simulink model "L2"  (R2023b)
settings: Solver=VariableStepAuto  StartTime=0.0  StopTime=50  RelTol=1e-3
undefined symbols (not defined in the file): b1, b2, k1, k2, m1, m2
settings Model: Creator=TRAN HUY LONG  LastModifiedBy=TRAN HUY LONG

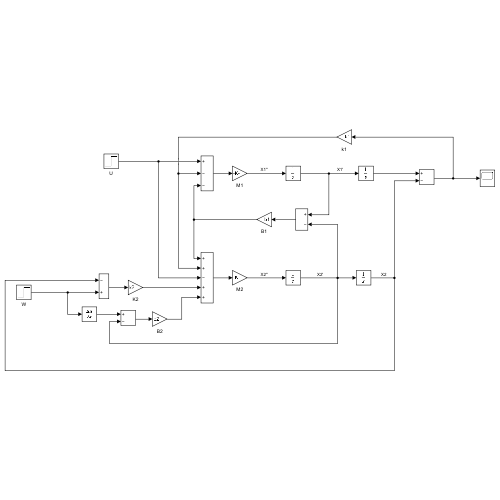
[thumbnail: Simulink's stored preview of the top-level diagram]
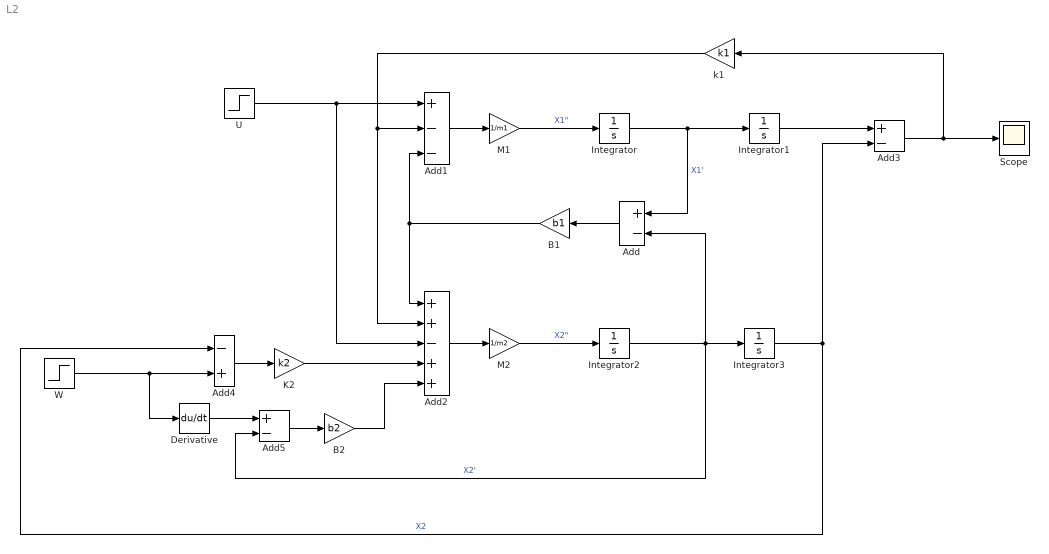
== system L2 ==
  Add : Sum  Inputs=+-
  Add1 : Sum  Inputs=+--
  Add2 : Sum  Inputs=++-++
  Add3 : Sum  Inputs=+-
  Add4 : Sum  Inputs=-+
  Add5 : Sum  Inputs=+-
  B1 : Gain  Gain=b1
  B2 : Gain  Gain=b2
  Derivative : Derivative
  Integrator{,1..3} (4 alike) : Integrator
  K2 : Gain  Gain=k2
  M1 : Gain  Gain=1/m1
  M2 : Gain  Gain=1/m2
  Scope : Scope
  U : Step  Time=0  OutDataTypeStr=Inherit: Inherit via back propagation  SampleTime=0
  W : Step  Time=0  After=0.1  OutDataTypeStr=Inherit: Inherit via back propagation  SampleTime=0
  k1 : Gain  Gain=k1
  wires:
  Integrator/1 -> Integrator1/1, Add/1  "X1'"
  M1/1 -> Integrator/1  "X1\""
  Integrator2/1 -> Add/2, Integrator3/1, Add5/2  "X2'"
  Integrator3/1 -> Add3/2, Add4/1  "X2"
  M2/1 -> Integrator2/1  "X2\""
  Add/1 -> B1/1
  Add1/1 -> M1/1
  B1/1 -> Add2/1, Add1/3
  k1/1 -> Add2/2, Add1/2
  U/1 -> Add2/3, Add1/1
  Add2/1 -> M2/1
  Integrator1/1 -> Add3/1
  Add3/1 -> k1/1, Scope/1
  K2/1 -> Add2/4
  Add4/1 -> K2/1
  W/1 -> Derivative/1, Add4/2
  Derivative/1 -> Add5/1
  Add5/1 -> B2/1
  B2/1 -> Add2/5
